simulink model "modelFedBatch"  (R2026a)
settings: Solver=VariableStepAuto  StopTime=14*3600
libraries: ChemReactorDesign_lib x8, nesl_utility x1
settings Model: Creator=klaus  LastModifiedBy=klaus
settings SolverCC: ZeroCrossAlgorithm=Adaptive
settings DebuggingCC: IgnoredZcDiagnostic=none
settings SimscapeCC: SimscapeNominalValues="[{\"value\":\"1\",\"unit\":\"A\"},{\"value\":\"1\",\"unit\":\"bar\"},{\"value\":\"1\",\"unit\":\"cm^2\"},{\"value\":\"1\",\"unit\":\"cm^3/s\"},{\"value\":\"1\",\"unit\":\"kJ/kg\"},{\"value\":\"1\",\"unit\":\"kW\"},{\"value\":\"1\",\"unit\":\"l\"},{\"value\":\"1\",\"unit\":\"N\"},{\"value\":\"1\",\"unit\":\"N*m\"},{\"value\":\"1\",\"unit\":\"V\"}]"  SimscapeLogDataHistory=5000.0  SimscapeCompileComponentReuse=on

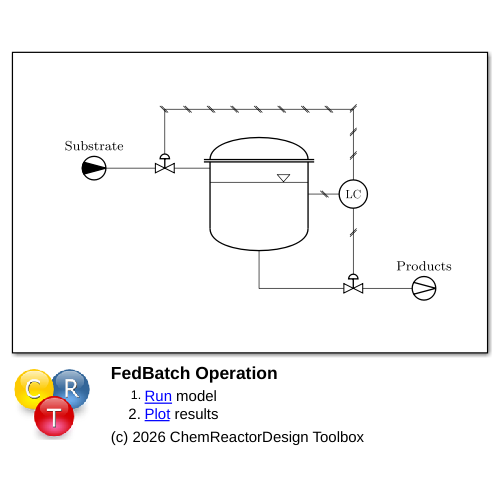
[thumbnail: Simulink's stored preview of the top-level diagram]
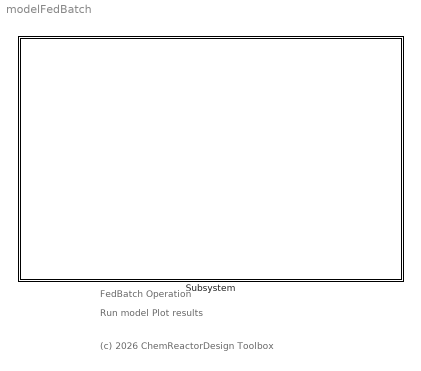
== system modelFedBatch ==
  note: Run model
      | Plot results
  note: FedBatch Operation
  note: (c) 2026 ChemReactorDesign Toolbox
  Subsystem : Subsystem

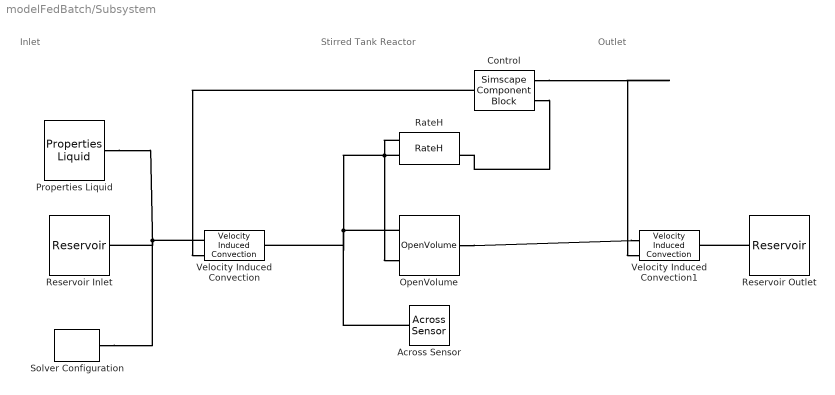
== system modelFedBatch/Subsystem ==
  note: Outlet
  note: Stirred Tank Reactor
  note: Inlet
  Across Sensor : ChemReactorDesign_lib/Basic/Liquid/Sensors/Across Sensor  concentrationsOutput=ChemReactorDesign.Basic.enum.OnOff.On  temperatureOutput=ChemReactorDesign.Basic.enum.OnOff.Off  pressureOutput=ChemReactorDesign.Basic.enum.OnOff.Off  fractionsOutput=ChemReactorDesign.Basic.enum.OnOff.Off  selectSpecies=[1, 2]
      settings: SourceProductName=Chemical Reactor Design ToolBox
  Control : SimscapeComponentBlock  SourceFile=FedBatchControl  ComponentPath=FedBatchControl  ComponentVariants="[\"FedBatchControl\"]"  ComponentVariantNames="[\"FedBatchControl\"]"  ClassName=FedBatchControl  SchemaVersion=1  Vmin=0.1 m^3  Vmax=1.2 m^3  isInput_specify=off  isInput_priority=None  isInput=1  isInput_nominal_specify=off  isInput_nominal_value=1  isInput_nominal_unit=1
      settings: CopyFcn=simscape.sscblock.internal.componentBlockCallback(gcbh,'COPY')  PreCopyFcn=simscape.sscblock.internal.componentBlockCallback(gcbh,'PRECOPY')  PreDeleteFcn=simscape.sscblock.internal.componentBlockCallback(gcbh,'PREDELETE')
      mask Type: FedBatchControl
  OpenVolume : ChemReactorDesign_lib/Basic/Liquid/Volumes/OpenVolume  pressureInput=ChemReactorDesign.Basic.enum.OnOff.Off  volumeOutput=ChemReactorDesign.Basic.enum.OnOff.On  hydrostaticPressure=ChemReactorDesign.Basic.enum.OnOff.Off  isothermalOperation=ChemReactorDesign.Basic.enum.OnOff.On  enable2ndPort=ChemReactorDesign.Basic.enum.OnOff.On  V0=0.1 m^3  A0=1 m^2  h0=0 m  x0=[0.0350262697022767 0.00175131348511384 0.963222416812609]  p0=1 bar  T0=298.15 K  n_nom=1 mol
      settings: SourceProductName=Chemical Reactor Design ToolBox
  Properties Liquid : ChemReactorDesign_lib/Basic/Liquid/Utilities/Properties Liquid  model=ChemReactorDesign.Basic.Liquid.enum.ThermodynamicModel.Ideal  N=3  Ids=[12;13;1]  Mw=[0;0;18.0153] g/mol  charge=[0;0;0]  table_T=[290 300] K  table_cp=[0 0 75.5402184579739;0 0 75.5425835956457] J/(K*mol)  table_Vm=[0 0 0.0180471322987256;0 0 0.018091238618091] l/mol  table_H=[0 0 -286.738719251556;0 0 -285.574694009364] kJ/mol  table_G=[0 0 -241.603407405;0 0 -239.651281374905] kJ/mol  table_mu=[0 0 0.00109430979865936;0 0 0.000860172426313474] Pa*s  table_lambda=[0 0 0.597518852340043;0 0 0.612989139138324] W/(K*m)  table_Hv=[0 0 44.3090602722826;0 0 43.9004472013488] kJ/mol  table_pvap=[0 0 1921.03049696876;0 0 3541.05430536848] Pa  A=[1 0 0;0 1 0;0 0 1] cal/mol  alpha=[0 0 0;0 0 0;0 0 0]  F_nom=1.0e-06 mol/s  Phi_nom=1.0 W  Q_nom=1.0 W  H_nom=1.0e+02 kJ/mol
      settings: SourceProductName=Chemical Reactor Design ToolBox
  RateH : ChemReactorDesign_lib/Basic/Liquid/Rates/RateH  rateReference=ChemReactorDesign.Basic.enum.RateReference.Volume  reversibility=ChemReactorDesign.Basic.enum.Reversibility.Irreversible  nu=[-1;1;0]  calculate_Ka=ChemReactorDesign.Basic.enum.OnOff.Off  Ka0=1.0e+30  kfinfV=0.8 mol/(hr*l)  kfinfA=0 mol/(cm^2*s)  kfinfm=0 mol/(g*s)  Ea=0 kJ/mol  kappaf=[1;1;0]  beta0=0.1  betainf=1  Es=0 kJ/mol  kappak=[1;0;0]  n=1
      settings: SourceProductName=Chemical Reactor Design ToolBox
  Reservoir Inlet : ChemReactorDesign_lib/Basic/Liquid/Utilities/Reservoir  x0=[0.0833333333333333 0 0.916666666666667]  p0=1 bar  T0=298.15 K
      settings: SourceProductName=Chemical Reactor Design ToolBox
  Reservoir Outlet : ChemReactorDesign_lib/Basic/Liquid/Utilities/Reservoir  x0=[0;0;1]  p0=1 bar  T0=298.15 K
      settings: SourceProductName=Chemical Reactor Design ToolBox
  Solver Configuration : nesl_utility/Solver Configuration  PhysicalDomain=network_engine_domain  SubClassName=solver  LeftPortType=input  RightPortType=generic  Tones=[]  Harmonics=[]  SimulateNoise=off  Profile=off  UseLocalSampling=off  EnableSwitchedLinearOptims=on  FrequencyDomain=off  UseCCode=off  RelTol=0.001  AbsTol=0.001  MinStep=1e-09  ToWorkspace=off  RevertToSquareIcSolve=off  NumHomotopyIterations=100  PhasorMode=off  PhasorModeNumHarmonics=1  ConsistencySolver=NEWTON_XTOL_AFTER_FTOL  CanonicalOrdering=UNORDERED  OptimizeIntermediates=UNOPTIMIZED  IndexReductionMethod=DerivativeReplacement  DoDC=off  ResidualTolerance=1e-09  ConsistencyTolSource=GLOBAL  ConsistencyAbsTol=0.001  ConsistencyRelTol=0.001  ConsistencyTolFactor=0.001  UseLocalSolver=off  LocalSolverChoice=NE_BACKWARD_EULER_ADVANCER  ResolveIndetEquations=on  FunctionEvalNumThread=1  LocalSolverSampleTime=0.001  DoFixedCost=off  MaxNonlinIter=3  MaxModeIter=2  ComputeImpulses=off  ImpulseIterations=2  LinearAlgebra=auto  LinearAlgebraNumThread=0  EquationFormulation=NE_TIME_EF  DelaysMemoryBudget=1024  AutomaticFiltering=on  FilteringTimeConstant=0.001  PartitionStorageMethod=AS_NEEDED  PartitionMemoryBudget=1024  PartitionMethod=ROBUST  MultibodyUseLocalSolver=off  MultibodyLocalSolverChoice=ODE1  MultibodyLocalSolverSampleTime=0.001
  Velocity Induced Convection : ChemReactorDesign_lib/Basic/Liquid/Transport/Velocity Induced Convection  flowInput=ChemReactorDesign.Basic.enum.OnOff.Off  controlInput=ChemReactorDesign.Basic.enum.OnOff.On  q0=0.1 m^3/hr  areaInput=ChemReactorDesign.Basic.enum.OnOff.Off  A0=1 m^2  delta=1.0e-03 m  flowOutput=ChemReactorDesign.Basic.enum.OnOff.Off  checkValve=ChemReactorDesign.Basic.enum.OnOff.Off  ymin=1.0e-10  q_specify=off  q_priority=None  q=0 l/s  q_nominal_specify=off  q_nominal_value=1  q_nominal_unit=l/s
      settings: SourceProductName=Chemical Reactor Design ToolBox
  Velocity Induced Convection1 : ChemReactorDesign_lib/Basic/Liquid/Transport/Velocity Induced Convection  flowInput=ChemReactorDesign.Basic.enum.OnOff.Off  controlInput=ChemReactorDesign.Basic.enum.OnOff.On  q0=0.4 m^3/hr  areaInput=ChemReactorDesign.Basic.enum.OnOff.Off  A0=1 m^2  delta=1.0e-03 m  flowOutput=ChemReactorDesign.Basic.enum.OnOff.Off  checkValve=ChemReactorDesign.Basic.enum.OnOff.Off  ymin=1.0e-10  q_specify=off  q_priority=None  q=0 l/s  q_nominal_specify=off  q_nominal_value=1  q_nominal_unit=l/s
      settings: SourceProductName=Chemical Reactor Design ToolBox
  connections:
  Velocity Induced Convection/LConn1 -- Solver Configuration/RConn1 -- Properties Liquid/RConn1 -- Reservoir Inlet/LConn1
  RateH/LConn2 -- Control/RConn2 -- OpenVolume/LConn2
  Reservoir Outlet/LConn1 -- Velocity Induced Convection1/RConn1
  OpenVolume/LConn1 -- RateH/LConn1 -- Velocity Induced Convection/RConn1 -- Across Sensor/LConn1
  OpenVolume/RConn1 -- Velocity Induced Convection1/LConn1
  Control/RConn1 -- Velocity Induced Convection1/LConn2
  Control/LConn1 -- Velocity Induced Convection/LConn2
